simulink model "super_regen_2"  (Simulink 7.4)
settings: Solver=ode45  StartTime=0.0  StopTime=8/1000  MaxStep=1/(5*Fcarrier)  RelTol=1e-3
PreLoadFcn:
  | Fcarrier=10e6;
  | C = 50e-12;
  | R = 1000;        % tank loss
  | Fmod=500;      % modulation freq
libraries: powerlib x7, simulink x4, dsparch4 x1, simulink_extras x1
settings Model: Creator=Dick Benson  LastModifiedBy=Dick
settings OptimizationCC: InitFltsAndDblsToZero=on

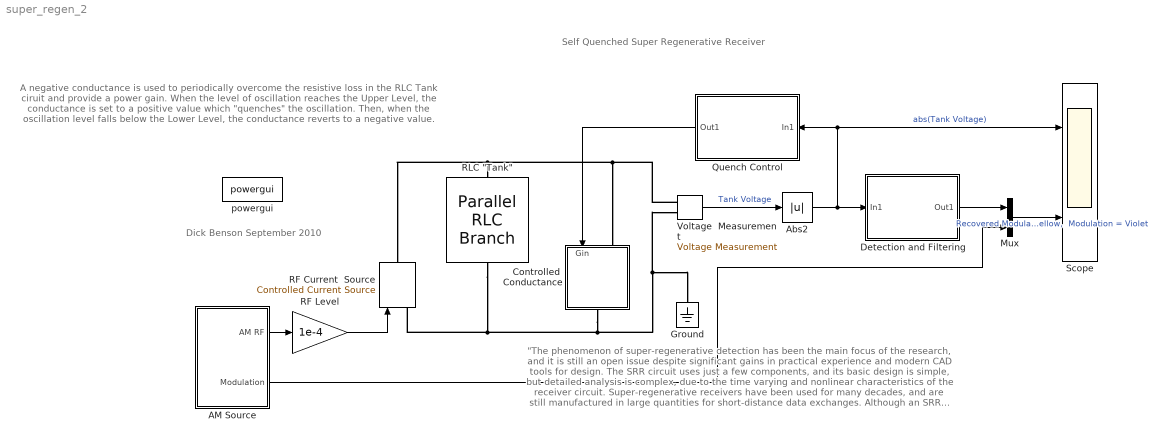
== system super_regen_2 ==
  note: Self Quenched Super Regenerative Receiver
  note: "The phenomenon of super-regenerative detection has been the main focus
      | of the research, and it is still an open issue despite significant gains in practical
      | experience and modern CAD tools for design. The SRR circuit uses just a few
      | components, and its basic design is simple, but detailed analysis is complex, due to the
      | time varying and nonlinear characteristics of the receiver circuit.
      | Super-regenerative receivers have been used for many decades, and are still
      | manufactured in large quantities for short-distance data exchanges. Although an SRR has
      | advantages of high gain, simplicity, low cost, low power consumption and constant
      | demodulated output over a wide range of input signal levels, it has also drawbacks of
      | inherent frequency instability."
      |
      | U.L. Rohde and A.K. Poddar, Synergy Microwave Corp., Paterson, NJ
      | http://www.mwjournal.com/BGDownload/Synergy_super_regenerative_receivers.pdf
  note: A negative conductance is used to periodically
      | overcome the resistive loss in the RLC Tank ciruit and provide a power gain.
      | When the level of oscillation reaches the Upper Level,
      | the conductance is set to a positive value which "quenches"
      | the oscillation. Then, when the oscillation level falls below
      | the Lower Level, the conductance reverts to a negative value.
  note: Dick Benson
      | September 2010
  AM Source : Subsystem
  Abs2 : Abs  OutDataType=sfix(16)  OutScaling=2^0
  Controlled  Conductance : Subsystem
  "Detection and Filtering " : Subsystem
  Ground : powerlib/Elements/Ground  DialogController=POWERSYS.PowerSysDialog  PhysicalDomain=powersysdomain  SubClassName=unknown  LeftPortType=p1  RightPortType=p1  LConnTagsString=a
  Mux : Mux  Inputs=2
  Quench Control : Subsystem
  RF Current  Source : powerlib/Electrical Sources/Controlled Current Source  DialogController=POWERSYS.PowerSysDialog  SystemSampleTime=-1  Initialize=on  Source_Type=DC  Amplitude=0  Phase=0  Frequency=0  Measurements=None
  RF Level : Gain  Gain=1e-4  ParameterDataType=sfix(16)  ParameterScaling=2^0  OutDataType=sfix(16)  OutScaling=2^0
  "RLC \"Tank\"" : powerlib/Elements/Parallel RLC Branch  DialogController=POWERSYS.PowerSysDialog  PhysicalDomain=powersysdomain  SubClassName=unknown  LeftPortType=p1  RightPortType=p1  LConnTagsString=a  RConnTagsString=__new0  BranchType=RLC  Resistance=R  Inductance=1/(((2*pi*Fcarrier)^2) *C)  SetiL0=off  InitialCurrent=0  Capacitance=C  Setx0=off  InitialVoltage=0  Measurements=None
  Scope : Scope  NumInputPorts=2
      settings: TimeRange=0.008  YMin=0~-4  YMax=4~6  MaxDataPoints=1e6
  Voltage  Measurement : powerlib/Measurements/Voltage Measurement  DialogController=POWERSYS.PowerSysDialog  SystemSampleTime=-1  PhasorSimulation=off  OutputType=Complex  PSBequivalent=0
  powergui : powerlib/powergui  SystemSampleTime=-1  SimulationMode=Continuous  SampleTime=50e-6  frequency=60  SPID=off  DisableSnubberDevices=off  DisableRonSwitches=off  DisableVfSwitches=off  SwTol=0  Interpol=off  frequencyindice=0  echomessages=off  HookPort=off  DisplayEquations=off  FunctionMessages=off  EnableUseOfTLC=off  x0status=blocks  RestoreLinks=warning  Frange=[0:2:500]  Ylog=off  Xlog=on  ShowGrid=off  save=off  variable=ZData  ZoomFFT=on  StartTime=0.0  cycles=1  DisplayStyle=1  fundamental=60  FreqAxis=off  MaxFrequency=1000  frequencyindicesteady=1  RmsSteady=1  display=off  Ts=0  methode=off
  wires:
  Quench Control/1(Out1) -> Controlled  Conductance/1(Gin)
  RF Level/1 -> RF Current  Source/1
  AM Source/2(Modulation) -> Mux/2
  AM Source/1(AM RF) -> RF Level/1
  Mux/1 -> Scope/2  "Recovered Modulation=Yellow,  Modulation = Violet"
  "Detection and Filtering "/1(Out1) -> Mux/1
  Voltage  Measurement/1 -> Abs2/1  "Tank Voltage"
  Abs2/1 -> Quench Control/1(In1), Scope/1, "Detection and Filtering "/1(In1)  "abs(Tank Voltage)"
  connections:
  Voltage  Measurement/LConn1 -- RF Current  Source/RConn1 -- "RLC \"Tank\""/LConn1 -- Controlled  Conductance/LConn1
  Voltage  Measurement/LConn2 -- Ground/LConn1 -- RF Current  Source/LConn1 -- "RLC \"Tank\""/RConn1 -- Controlled  Conductance/RConn1

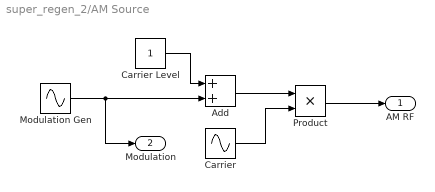
== system super_regen_2/AM Source ==
  Add : Sum  OutDataType=sfix(16)  OutScaling=2^-10
  Carrier : Sin  Amplitude=1  Bias=0  Frequency=Fcarrier*2*pi  Phase=0  Samples=10  SampleTime=0  Offset=0
  Carrier Level : Constant  OutDataType=sfix(16)  OutScaling=2^0
  Modulation Gen : Sin  Amplitude=1  Bias=0  Frequency=Fmod*2*pi  Phase=0  Samples=10  SampleTime=0  Offset=0
  Product : Product  OutDataType=sfix(16)  OutScaling=2^0  RndMeth=Zero
  AM RF : Outport
  Modulation : Outport  Port=2
  wires:
  Modulation Gen/1 -> Add/2, Modulation/1
  Carrier/1 -> Product/2
  Product/1 -> AM RF/1
  Carrier Level/1 -> Add/1
  Add/1 -> Product/1

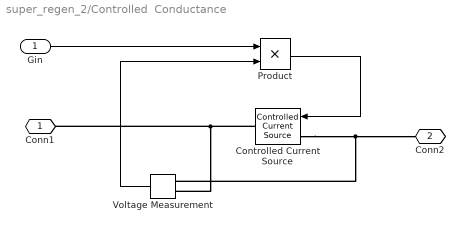
== system super_regen_2/Controlled  Conductance ==
  Gin : Inport  OutDataType=sfix(16)  OutScaling=2^0
  Controlled Current Source : powerlib/Electrical Sources/Controlled Current Source  DialogController=POWERSYS.PowerSysDialog  SystemSampleTime=-1  Initialize=on  Source_Type=AC  Amplitude=0  Phase=0  Frequency=0  Measurements=None
  Product : Product  OutDataType=sfix(16)  OutScaling=2^0  RndMeth=Zero
  Voltage Measurement : powerlib/Measurements/Voltage Measurement  DialogController=POWERSYS.PowerSysDialog  SystemSampleTime=-1  PhasorSimulation=off  OutputType=Complex  PSBequivalent=0
  Conn1 : PMIOPort  Port=1  Side=Left
  Conn2 : PMIOPort  Port=2  Side=Right
  wires:
  Gin/1 -> Product/1
  Product/1 -> Controlled Current Source/1
  Voltage Measurement/1 -> Product/2
  connections:
  Controlled Current Source/LConn1 -- Conn2/RConn1 -- Voltage Measurement/LConn1
  Controlled Current Source/RConn1 -- Conn1/RConn1 -- Voltage Measurement/LConn2

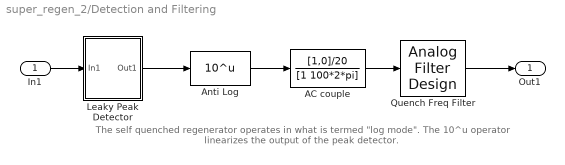
== system super_regen_2/Detection and Filtering  ==
  note: The self quenched regenerator operates in what is termed "log mode".
      | The 10^u operator linearizes the output of the peak detector.
  In1 : Inport
  AC couple : TransferFcn  Numerator=[1,0]/20  Denominator=[1 100*2*pi]
  Anti Log : Math  Operator=10^u  OutDataType=fixdt(1, 16)  OutScaling=2^0  SaturateOnIntegerOverflow=on
  Leaky Peak Detector : Subsystem
  "Quench Freq Filter " : dsparch4/Analog Filter Design  method=Elliptic  filttype=Lowpass  N=3  Wlo=4000*2*pi  Whi=80  Rp=1  Rs=60
  Out1 : Outport
  wires:
  Leaky Peak Detector/1(Out1) -> Anti Log/1
  Anti Log/1 -> AC couple/1
  AC couple/1 -> "Quench Freq Filter "/1
  In1/1 -> Leaky Peak Detector/1(In1)
  "Quench Freq Filter "/1 -> Out1/1

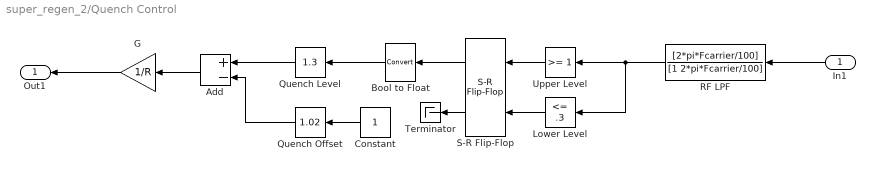
== system super_regen_2/Quench Control ==
  In1 : Inport
  Add : Sum  Inputs=+-  OutDataType=sfix(16)  OutScaling=2^-10
  Bool to Float : DataTypeConversion  OutDataType=fixdt(1, 16)  OutScaling=2^0
  Constant : Constant  OutDataType=sfix(16)  OutScaling=2^0
  G : Gain  Gain=1/R  ParameterDataType=sfix(16)  ParameterScaling=2^0  OutDataType=sfix(16)  OutScaling=2^0
  Lower Level : simulink/Logic and Bit Operations/Compare To Constant  SystemSampleTime=-1  relop=<=  const=.3  LogicOutDataTypeMode=boolean
  Quench Level : simulink/Math Operations/Slider Gain  SystemSampleTime=-1  low=0  gain=1.3  high=2
  Quench Offset : simulink/Math Operations/Slider Gain  SystemSampleTime=-1  low=0.9  gain=1.02  high=1.1
  RF LPF : TransferFcn  Numerator=[2*pi*Fcarrier/100]  Denominator=[1 2*pi*Fcarrier/100]
  S-R Flip-Flop : simulink_extras/Flip Flops/S-R Flip-Flop  SystemSampleTime=-1  initial_condition=0
  Terminator : Terminator
  Upper Level : simulink/Logic and Bit Operations/Compare To Constant  SystemSampleTime=-1  relop=>=  const=1  LogicOutDataTypeMode=boolean
  Out1 : Outport
  wires:
  Constant/1 -> Quench Offset/1
  Bool to Float/1 -> Quench Level/1
  S-R Flip-Flop/1 -> Bool to Float/1
  Upper Level/1 -> S-R Flip-Flop/1
  Lower Level/1 -> S-R Flip-Flop/2
  RF LPF/1 -> Upper Level/1, Lower Level/1
  Quench Level/1 -> Add/1
  Quench Offset/1 -> Add/2
  In1/1 -> RF LPF/1
  Add/1 -> G/1
  S-R Flip-Flop/2 -> Terminator/1
  G/1 -> Out1/1

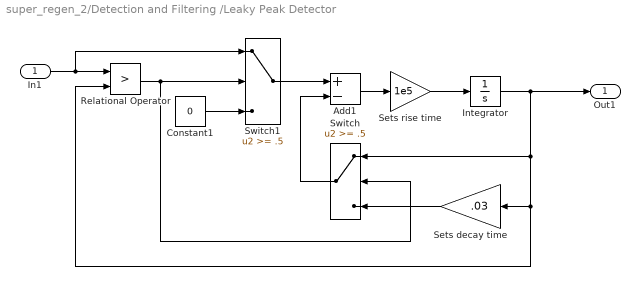
== system super_regen_2/Detection and Filtering /Leaky Peak Detector ==
  In1 : Inport
  Add1 : Sum  Inputs=+-  OutDataType=sfix(16)  OutScaling=2^-10
  Constant1 : Constant  Value=0  OutDataType=sfix(16)  OutScaling=2^0
  Integrator : Integrator
  Relational Operator : RelationalOperator  Operator=>  LogicOutDataTypeMode=boolean  LogicDataType=fixdt(0, 8)  OutDataTypeStr=boolean
  Sets decay time : Gain  Gain=.03  ParameterDataType=fixdt(1, 16)  ParameterScaling=2^0  OutDataType=fixdt(1, 16)  OutScaling=2^0
  Sets rise time : Gain  Gain=1e5  ParameterDataType=fixdt(1, 16)  ParameterScaling=2^0  OutDataType=fixdt(1, 16)  OutScaling=2^0
  Switch : Switch  Threshold=.5  OutDataType=fixdt(1, 16)  OutScaling=2^0
  Switch1 : Switch  Threshold=.5  OutDataType=fixdt(1, 16)  OutScaling=2^0
  Out1 : Outport  OutDataType=fixdt(1, 16)  OutScaling=2^0
  wires:
  Add1/1 -> Sets rise time/1
  Integrator/1 -> Switch/1, Sets decay time/1, Relational Operator/2, Out1/1
  Sets rise time/1 -> Integrator/1
  Sets decay time/1 -> Switch/3
  Switch/1 -> Add1/2
  Relational Operator/1 -> Switch/2, Switch1/2
  Switch1/1 -> Add1/1
  Constant1/1 -> Switch1/3
  In1/1 -> Relational Operator/1, Switch1/1
